simulink model "kalmanTest"  (R2014a)
settings: Solver=ode45  StartTime=0.0  StopTime=1  RelTol=1e-3
values from neighbouring files (symbols this model uses):
  dz = [ 0.1; -0.1; -0.1; 0.1]    [KF_testScript.m]
  dz_r = sin(pi/6)*[ 0.01; -0.01; -0.01; 0.01]    [KF_testScript.m]
  f_r = [0.1; 0.05]    [KF_testScript.m]
  x_check = zeros(9,1)    [KF_testScript.m]
  x_check_r = [psi_r; v_r; p_r]    [KF_testScript.m]
undefined symbols (not defined in the file or in its folder): kalman_r
settings Model: Creator=mariutho  LastModifiedBy=mariutho

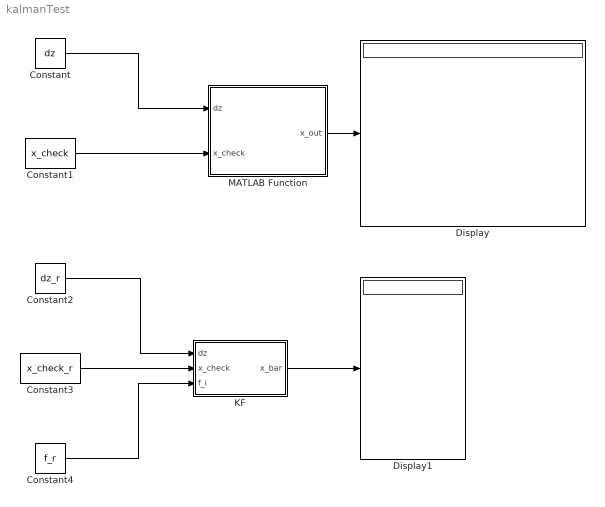
== system kalmanTest ==
  Constant : Constant  Value=dz
  Constant1 : Constant  Value=x_check
  Constant2 : Constant  Value=dz_r
  Constant3 : Constant  Value=x_check_r
  Constant4 : Constant  Value=f_r
  Display : Display
  Display1 : Display
  KF : Subsystem
  MATLAB Function : MATLAB Function  TreatAsAtomicUnit=on
  wires:
  Constant/1 -> MATLAB Function/1(dz)
  Constant1/1 -> MATLAB Function/2(x_check)
  MATLAB Function/1(x_out) -> Display/1
  Constant2/1 -> KF/1(dz)
  Constant3/1 -> KF/2(x_check)
  KF/1(x_bar) -> Display1/1
  Constant4/1 -> KF/3(f_i)

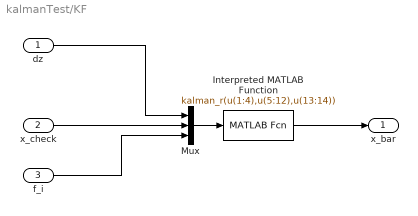
== system kalmanTest/KF ==
  dz : Inport
  x_check : Inport  Port=2
  f_i : Inport  Port=3
  Interpreted MATLAB Function : MATLABFcn  MATLABFcn=kalman_r(u(1:4),u(5:12),u(13:14))
  Mux : Mux  Inputs=3
  x_bar : Outport
  wires:
  Interpreted MATLAB Function/1 -> x_bar/1
  x_check/1 -> Mux/2
  dz/1 -> Mux/1
  Mux/1 -> Interpreted MATLAB Function/1
  f_i/1 -> Mux/3

== matlab function kalmanTest/MATLAB Function ==
  data: dz input; x_out output; x_check input
function x_out = kalman(dz, x_check)
% 	persistent x;
% 	N = length(dz)/2;
% 	% state vector
% 	% [dpsi, dv, dp, b_a, b_g]'
% 	
% 	x_out = zeros(N,1);
%     persistent P x_est H Q R x_pred
% 	
% 	% Initialization
%     if isempty(P)
%         % First time through the code so do some initialization
%         x_est = zeros(N,1);
% 		x_pred = zeros(N,1);
%         P = zeros(N);
%         
%         H = e;
%         Q = 0.01*eye(N);
%         R = eye(6);
%     end
%     % Propagate the state estimate and covariance matrix:
% 	% Time update
%   	%[T,Y] = ode23('dynamics',[0 0.01],[x_est;tau; zeros(3,1)]);
%   	x_pred = Y(length(T),1:6)';
%  	
%  	F = lin3DOF(x_est);
%   	sys = ss(F,B,H,0);
%   	sysd = c2d(sys,0.01);
% 	Ad = sysd.a;
%  	P = Ad*P*Ad' + Q;
% 
% 	% Update the state and error covariance estimate
% 	% Measurment update
% 	% Calculate the Kalman gain
% 	K = P*H'/(H*P*H' + R);
%     x_est = x_pred + K*(y - H*x_pred);
%     P = (eye(size(K,1))-K*H)*P;
%     % Post the results
% 	x_out = x_est;
	x_out = -1;
end
